simulink model "closedloop_enlarged_initialstates"  (R2021a)
settings: Solver=ode15s  StartTime=0.0  StopTime=75  RelTol=1e-7  AbsTol=1e-7  EnableMultiTasking=on
InitFcn:
  | datacstr
undefined symbols (not defined in the file or in its folder): c_bar, cp, cstrfun, DH, ER, eta_bar, Ken_eta, Ken_x, ko, q, r, T_bar, Tf, UA, V
settings Model: ExtModeTrigMode=oneshot  ExtModeArmWhenConnect=off  Creator=scattolini  LastModifiedBy=fabio
settings SolverCC: AutoScaleAbsTol=off  AlgebraicLoopSolver=TrustRegion
settings DataIOCC: SaveFormat=Array  SignalLoggingSaveFormat=ModelDataLogs  ReturnWorkspaceOutputs=off  SignalLoggingName=sigsOut
settings OptimizationCC: BlockReduction=off  BooleanDataType=off  DefaultParameterBehavior=Inlined  BufferReuse=off  ExpressionDepthLimit=2147483647  InitFltsAndDblsToZero=on  LifeSpan=inf
settings DebuggingCC: SaveWithParameterizedLinksMsg=none  UnderspecifiedInitializationDetection=Classic  MergeDetectMultiDrivingBlocksExec=none  SignalResolutionControl=TryResolveAllWithWarning  MultiTaskDSMMsg=warning  MultiTaskCondExecSysMsg=none  FcnCallInpInsideContextMsg=warning  StateNameClashWarn=warning  SFUnexpectedBacktrackingDiag=warning  SFNoUnconditionalDefaultTransitionDiag=warning  SFExecutionAtInitializationDiag=none  SFMachineParentedDataDiag=warning  ArithmeticOperatorsInVariantConditions=warning
settings HardwareCC: ProdBitPerPointer=32  ProdBitPerSizeT=32  ProdBitPerPtrDiffT=32  ProdLargestAtomicFloat=None  ProdIntDivRoundTo=Undefined  ProdEndianess=Unspecified  ProdWordSize=32  ProdHWDeviceType=32-bit Generic  TargetUnknown=on
settings ModelReferenceCC: PropagateSignalLabelsOutOfModel=off
settings SFSimCC: SimUseLocalCustomCode=off  CustomCodeUndefinedFunction=UseInterfaceOnly
settings RTWCC: Description=Generic Real-Time Target  RTWUseLocalCustomCode=off
settings CodeAppCC: StateflowObjectComments=on
settings GRTTargetCC: TargetFcnLib=ansi_tfl_tmw.mat  TargetLangStandard=C89/C90 (ANSI)  CombineOutputUpdateFcns=off  GRTInterface=on
settings ConfigComp: CovMetricSettings=dw  CovSaveCumulativeToWorkspaceVar=on  CovSaveSingleToWorkspaceVar=on  CovExternalEMLEnable=off  CovSFcnEnable=off

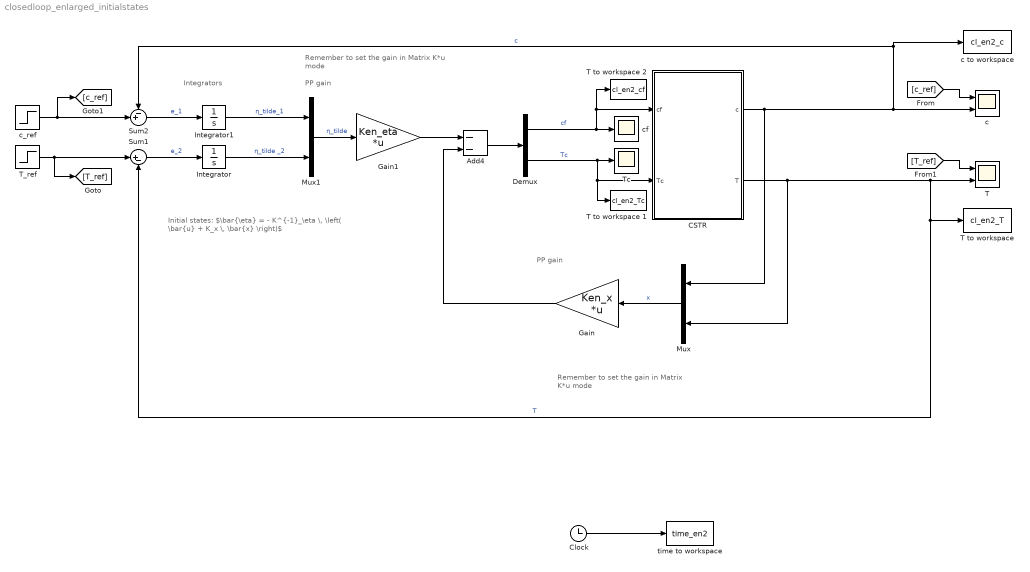
== system closedloop_enlarged_initialstates ==
  note: PP gain
  note: PP gain
  note: Integrators
  note: Remember to set the gain in
      | Matrix K*u mode
  note: Remember to set the gain in
      | Matrix K*u mode
  note: Initial states:
      | $\bar{\eta} = - K^{-1}_\eta \, \left( \bar{u} + K_x \, \bar{x} \right)$
  Add4 : Sum  Inputs=--
  CSTR : Subsystem
  Clock : Clock
  Demux : Demux  Outputs=2
  Gain : Gain  Gain=Ken_x  Multiplication=Matrix(K*u) (u vector)
  Gain1 : Gain  Gain=Ken_eta  Multiplication=Matrix(K*u) (u vector)
  Integrator : Integrator  InitialCondition=eta_bar(2)
  Integrator1 : Integrator  InitialCondition=eta_bar(1)
  Mux : Mux  Inputs=2
  Mux1 : Mux  Inputs=2
  Sum1 : Sum  Inputs=|+-
  Sum2 : Sum  Inputs=-+|
  T : Scope  NumInputPorts=2
  "T to workspace " : ToWorkspace  VariableName=cl_en2_T  SampleTime=-1
  T to workspace 1 : ToWorkspace  VariableName=cl_en2_Tc  SampleTime=-1
  T to workspace 2 : ToWorkspace  VariableName=cl_en2_cf  SampleTime=-1
  T_ref : Step  Time=30  Before=350  After=340  SampleTime=0
  Tc : Scope
  c : Scope  NumInputPorts=2
  "c to workspace " : ToWorkspace  VariableName=cl_en2_c  SampleTime=-1
  c_ref : Step  Time=10  Before=0.5  After=0.55  SampleTime=0
  cf : Scope
  time to workspace : ToWorkspace  VariableName=time_en2  SampleTime=-1
  wires:
  Clock/1 -> time to workspace/1
  CSTR/1(c) -> Mux/1, c/2, "c to workspace "/1, Sum2/1  "c"
  Mux/1 -> Gain/1  "x"
  Integrator1/1 -> Mux1/1  "η_tilde_1"
  Integrator/1 -> Mux1/2  "η_tilde _2"
  Sum1/1 -> Integrator/1  "e_2"
  c_ref/1 -> [c_ref], Sum2/2
  T_ref/1 -> [T_ref], Sum1/1
  Gain/1 -> Add4/2
  Add4/1 -> Demux/1
  CSTR/2(T) -> Mux/2, Sum1/2, "T to workspace "/1, T/2  "T"
  Mux1/1 -> Gain1/1  "η_tilde"
  Sum2/1 -> Integrator1/1  "e_1"
  Gain1/1 -> Add4/1
  [c_ref] -> c/1
  [T_ref] -> T/1
  Demux/1 -> T to workspace 2/1, CSTR/1(cf), cf/1  "cf"
  Demux/2 -> T to workspace 1/1, CSTR/2(Tc), Tc/1  "Tc"

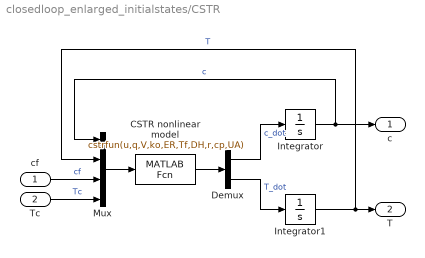
== system closedloop_enlarged_initialstates/CSTR ==
  cf : Inport  PortDimensions=1
  Tc : Inport  Port=2  PortDimensions=1
  CSTR nonlinear model : MATLABFcn  MATLABFcn=cstrfun(u,q,V,ko,ER,Tf,DH,r,cp,UA)  OutputDimensions=2
  Demux : Demux  Outputs=2
      settings: DisplayOption=none
  Integrator : Integrator  InitialCondition=c_bar + 0.025
  Integrator1 : Integrator  InitialCondition=T_bar + 2.5
  Mux : Mux
  c : Outport  PortDimensions=1
  T : Outport  Port=2  PortDimensions=1
  wires:
  Mux/1 -> CSTR nonlinear model/1
  CSTR nonlinear model/1 -> Demux/1
  Demux/1 -> Integrator/1  "c_dot"
  Demux/2 -> Integrator1/1  "T_dot"
  Integrator1/1 -> Mux/2, T/1  "T"
  Integrator/1 -> Mux/1, c/1  "c"
  cf/1 -> Mux/3  "cf"
  Tc/1 -> Mux/4  "Tc"
